simulink model "UdpClient"  (R2016b)
settings: Solver=FixedStepDiscrete  StartTime=0.0  StopTime=inf  FixedStep=CassieParameters.etherCatSampleTime  RelTol=1e-3  EnableMultiTasking=on
InitFcn:
  | udpInitFcn;
undefined symbols (not defined in the file or in its folder): inputBytes, outputBytes
libraries: ptplib x3, xpcutilitieslib x2
settings Model: xpc_rtwmakecfg_data=_xpciplib__xpcetherlib__xpcether8255xlib__xpcetherGbElib__xpcnblib_  SimulationMode=external  Creator=robot  LastModifiedBy=mikha
settings SolverCC: EnableConcurrentExecution=on
settings DataIOCC: SaveFormat=Array  SaveOutput=off  SignalLogging=off  DSMLogging=off  VisualizeSimOutput=off  SaveTime=off
settings OptimizationCC: DefaultParameterBehavior=Inlined  OptimizeBlockIOStorage=off  BufferReuse=off  GlobalBufferReuse=off  ExpressionFolding=off  LocalBlockOutputs=off  LifeSpan=inf  SimCompilerOptimization=on  AccelVerboseBuild=on
settings DebuggingCC: AllowSymbolicDim=off  SFUnexpectedBacktrackingDiag=warning  SFNoUnconditionalDefaultTransitionDiag=warning  SFExecutionAtInitializationDiag=none
settings HardwareCC: ProdBitPerPointer=32  ProdBitPerSizeT=32  ProdBitPerPtrDiffT=32  ProdLargestAtomicFloat=None  ProdWordSize=32  ProdLongLongMode=on  ProdHWDeviceType=Generic->32-bit x86 compatible
settings ModelReferenceCC: EnableParallelModelReferenceBuilds=on  ParallelModelReferenceMATLABWorkerInit=Copy Base Workspace  ModelReferenceNumInstancesAllowed=Zero  PropagateSignalLabelsOutOfModel=off
settings SFSimCC: SFSimEcho=off
settings RTWCC: SystemTargetFile=slrt.tlc  TLCOptions=-axPCMaxOverloads=1000000000 -axPCMaxOverloadLen=1000000000  TemplateMakefile=slrt_default_tmf  Description=Simulink Real-Time  RTWCompilerOptimization=on
settings CodeAppCC: GenerateComments=off  SimulinkBlockComments=off
settings ConfigComp: CovMetricSettings=dw  CovHtmlReporting=on  CovSaveCumulativeToWorkspaceVar=on  CovSaveSingleToWorkspaceVar=on  CovExternalEMLEnable=off

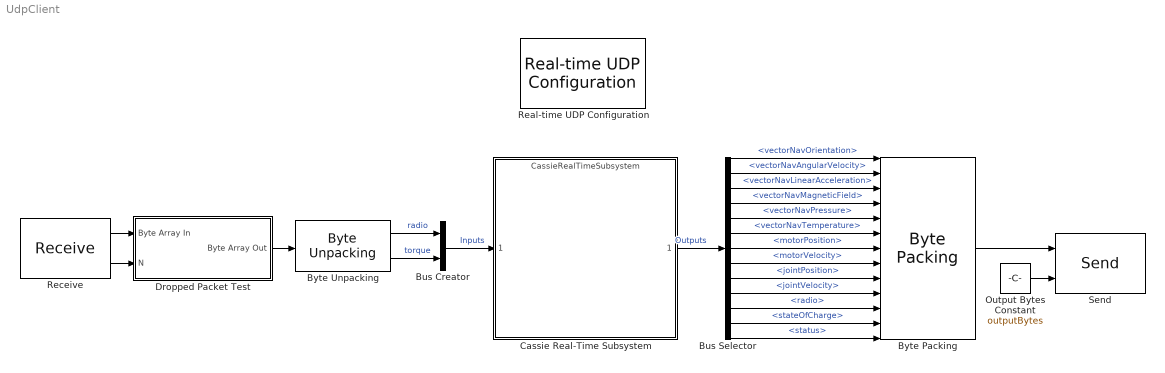
== system UdpClient ==
  Bus Creator : BusCreator  Inputs=2  OutDataTypeStr=Bus: cassieInputsBus
  Bus Selector : BusSelector  OutputSignals=vectorNavOrientation,vectorNavAngularVelocity,vectorNavLinearAcceleration,vectorNavMagneticField,vectorNavPressure,vectorNavTemperature,motorPosition,motorVelocity,jointPosition,jointVelocity,radio,stateOfCharge,status
  "Byte Packing " : xpcutilitieslib/Byte Packing   MaskPackedDataType=uint8  MaskUnpackedDataTypes=outputTypes  MaskAlignment=1
  "Byte Unpacking " : xpcutilitieslib/Byte Unpacking   MaskUnpackedDataTypes=inputTypes  MaskUnpackedDataSizes=inputSizes  MaskAlignment=1
  Cassie Real-Time Subsystem : ModelReference  ModelNameDialog=CassieRealTimeSubsystem  SimulationMode=Normal  ModelReferenceVersion=1.1267
      mask Display: image('Cassie.png');
  Dropped Packet Test : Subsystem  mask{timeWindow=500, droppedPacks=250}
      mask prompts: timeWindow "Time window (samples)"; droppedPacks "Dropped msg threshold"
      mask help: Tests UDP data for continuity. Time window specifies the duration of the running average in samples, and if the number of dropped messages is higher than Dropped msg threshold, the UDP inputs are set to zero
      mask init:
      | if timeWindow < droppedPacks
      |   error('Dropped message threshold must be lower than the Time Window')
      | end
  Output Bytes Constant : Constant  Value=outputBytes
  "Real-time UDP Configuration " : ptplib/PTP UDP/Real-time UDP  Configuration   ID=1  IpAddress=10.10.10.3  SubnetMask=255.255.255.0  Gateway=0.0.0.0  EthDrv=Intel Gigabit  PciBus=3  PciSlot=0  udpID=0  MulticastList=[]  Multicast={}
  "Receive " : ptplib/PTP UDP/Receive   ID=1  Receive1=0.0.0.0  Receive2=25001  Receive3=inputBytes  Receive4=-1  udpID=0
  "Send " : ptplib/PTP UDP/Send   ID=1  Send1=255.255.255.255  Send2=25000  Send3=-1  Send4=-1  udpID=0
  wires:
  "Byte Unpacking "/2 -> Bus Creator/2  "torque"
  "Byte Unpacking "/1 -> Bus Creator/1  "radio"
  Bus Creator/1 -> Cassie Real-Time Subsystem/1  "Inputs"
  Cassie Real-Time Subsystem/1 -> Bus Selector/1  "Outputs"
  Bus Selector/13 -> "Byte Packing "/13  "<status>"
  Bus Selector/12 -> "Byte Packing "/12  "<stateOfCharge>"
  Bus Selector/11 -> "Byte Packing "/11  "<radio>"
  Bus Selector/10 -> "Byte Packing "/10  "<jointVelocity>"
  Bus Selector/9 -> "Byte Packing "/9  "<jointPosition>"
  Bus Selector/8 -> "Byte Packing "/8  "<motorVelocity>"
  Bus Selector/7 -> "Byte Packing "/7  "<motorPosition>"
  Bus Selector/6 -> "Byte Packing "/6  "<vectorNavTemperature>"
  Bus Selector/4 -> "Byte Packing "/4  "<vectorNavMagneticField>"
  Bus Selector/3 -> "Byte Packing "/3  "<vectorNavLinearAcceleration>"
  Bus Selector/5 -> "Byte Packing "/5  "<vectorNavPressure>"
  Bus Selector/1 -> "Byte Packing "/1  "<vectorNavOrientation>"
  Bus Selector/2 -> "Byte Packing "/2  "<vectorNavAngularVelocity>"
  "Byte Packing "/1 -> "Send "/1
  "Receive "/1 -> Dropped Packet Test/1(Byte Array In)
  "Receive "/2 -> Dropped Packet Test/2(N)
  Dropped Packet Test/1(Byte Array Out) -> "Byte Unpacking "/1
  Output Bytes Constant/1 -> "Send "/2

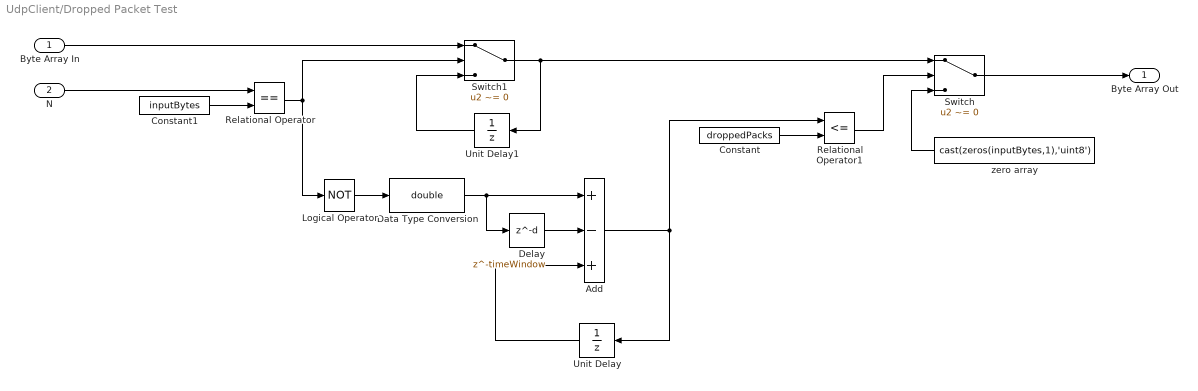
== system UdpClient/Dropped Packet Test ==
  Byte Array In : Inport
  N : Inport  Port=2
  Add : Sum  Inputs=+-+
  Constant : Constant  Value=droppedPacks
  Constant1 : Constant  Value=inputBytes
  Data Type Conversion : DataTypeConversion  OutDataTypeStr=double
  Delay : Delay  DelayLength=timeWindow
  Logical Operator : Logic  Operator=NOT  AllPortsSameDT=off  OutDataTypeStr=boolean
  Relational Operator : RelationalOperator  Operator===  OutDataTypeStr=boolean  RndMeth=Simplest
  Relational Operator1 : RelationalOperator  Operator=<=  OutDataTypeStr=boolean  RndMeth=Simplest
  Switch : Switch  Criteria=u2 ~= 0
  Switch1 : Switch  Criteria=u2 ~= 0
  Unit Delay : UnitDelay  SampleTime=-1
  Unit Delay1 : UnitDelay  SampleTime=-1
  zero array : Constant  Value=cast(zeros(inputBytes,1),'uint8')
  Byte Array Out : Outport
  wires:
  Relational Operator/1 -> Logical Operator/1, Switch1/2
  zero array/1 -> Switch/3
  Constant1/1 -> Relational Operator/2
  Logical Operator/1 -> Data Type Conversion/1
  Delay/1 -> Add/2
  Unit Delay/1 -> Add/3
  Add/1 -> Relational Operator1/1, Unit Delay/1
  Data Type Conversion/1 -> Add/1, Delay/1
  N/1 -> Relational Operator/1
  Switch/1 -> Byte Array Out/1
  Constant/1 -> Relational Operator1/2
  Relational Operator1/1 -> Switch/2
  Byte Array In/1 -> Switch1/1
  Switch1/1 -> Switch/1, Unit Delay1/1
  Unit Delay1/1 -> Switch1/3
